simulink model "vexv5_Clawbot_Driver_Safety"  (R2019a)
settings: Solver=ode3  StartTime=0.0  StopTime=inf  RelTol=1e-3  EnableMultiTasking=on
libraries: vexv5lib x9, vexcommonlib x1
settings Model: ExtModeTrigDuration=5  Creator=The MathWorks, Inc.  LastModifiedBy=josea
settings DataIOCC: LimitDataPoints=on  SaveFormat=Array  ReturnWorkspaceOutputs=off
settings OptimizationCC: ExpressionDepthLimit=2147483647  LifeSpan=Inf  MaxStackSize=64
settings DebuggingCC: UnderspecifiedInitializationDetection=Classic  MergeDetectMultiDrivingBlocksExec=none  InheritedTsInSrcMsg=none  FcnCallInpInsideContextMsg=warning  UnconnectedInputMsg=none  UnconnectedOutputMsg=none  AllowSymbolicDim=off  StateNameClashWarn=warning  SFUnexpectedBacktrackingDiag=warning  SFNoUnconditionalDefaultTransitionDiag=warning  SFExecutionAtInitializationDiag=none  ArithmeticOperatorsInVariantConditions=warning
settings HardwareCC: ProdBitPerPointer=32  ProdBitPerSizeT=32  ProdBitPerPtrDiffT=32  ProdLargestAtomicInteger=Long  ProdLargestAtomicFloat=Double  ProdWordSize=32  ProdHWDeviceType=ARM Compatible->ARM Cortex
settings ModelReferenceCC: PropagateSignalLabelsOutOfModel=off
settings SFSimCC: SimUseLocalCustomCode=off
settings RTWCC: SystemTargetFile=ert.tlc  HardwareBoard=VEX V5 Robot Brain  TLCOptions=-aInlineSetEventsForThisBaseRateFcn=TLC_FALSE -aSuppressMultiTaskScheduler=TLC_FALSE -aRateBasedStepFcn=0  TemplateMakefile=ert_default_tmf  RTWUseLocalCustomCode=off  Toolchain=GNU Tools for ARM Embedded Processors
settings CodeAppCC: StateflowObjectComments=on
settings ERTTargetCC: CodeReplacementLibrary=GCC ARM Cortex-M3  MultiwordLength=2048  ERTCustomFileBanners=off  SupportContinuousTime=on  SupportNonInlinedSFcns=on  RemoveResetFunc=off  ModelStepFunctionPrototypeControlCompliant=off  ConvertIfToSwitch=off  SuppressUnreachableDefaultCases=off
settings ConfigComp: CovMetricSettings=dw  CovHtmlReporting=on  CovSaveCumulativeToWorkspaceVar=on  CovSaveSingleToWorkspaceVar=on  CovExternalEMLEnable=off  CovSFcnEnable=off

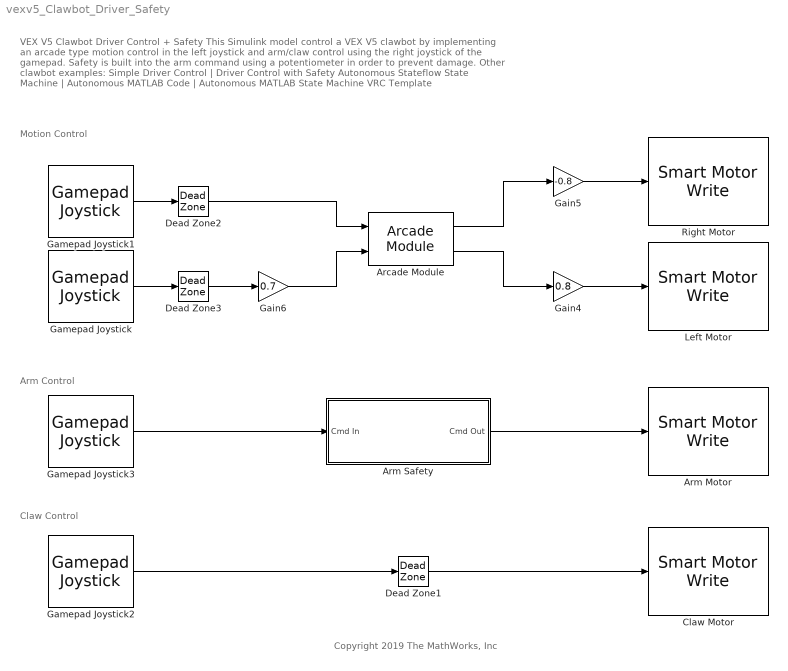
== system vexv5_Clawbot_Driver_Safety ==
  note: Claw Control
  note: Arm Control
  note: Motion Control
  note: Copyright 2019 The MathWorks, Inc
  note: VEX V5 Clawbot Driver Control + Safety
      | This Simulink model control a VEX V5 clawbot by implementing an arcade type motion control in the left joystick and arm/claw control using
      | the right joystick of the gamepad. Safety is built into the arm command using a potentiometer in order to prevent damage. Other clawbot examples:
      | Simple Driver Control | Driver Control with Safety
      | Autonomous Stateflow State Machine | Autonomous MATLAB Code | Autonomous MATLAB State Machine
      | VRC Template
  Arcade Module : vexcommonlib/Arcade Module  BlockPlatform=vexarmcortex
      settings: SourceProductName=Simulink Coder Support Package for ARM Cortex-based VEX Microcontroller  SourceProductBaseCode=EC_VEX_MICRO
  Arm Motor : vexv5lib/Actuators/Smart Motor Write  motorPort=8  scaleFactor=18:1  MotorBrakeMode=Hold  OperationMode=Velocity Control
      settings: SourceProductName=Simulink Coder Support Package for VEX EDR V5 Robot Brain
  Arm Safety : Subsystem
  Claw Motor : vexv5lib/Actuators/Smart Motor Write  motorPort=3  scaleFactor=18:1  MotorBrakeMode=Hold  OperationMode=Velocity Control
      settings: SourceProductName=Simulink Coder Support Package for VEX EDR V5 Robot Brain
  Dead Zone1 : DeadZone  LowerValue=-5  UpperValue=5  SaturateOnIntegerOverflow=on
  Dead Zone2 : DeadZone  LowerValue=-5  UpperValue=5  SaturateOnIntegerOverflow=on
  Dead Zone3 : DeadZone  LowerValue=-5  UpperValue=5  SaturateOnIntegerOverflow=on
  Gain4 : Gain  Gain=0.8
  Gain5 : Gain  Gain=-0.8
  Gain6 : Gain  Gain=0.7
  Gamepad Joystick : vexv5lib/Gamepad/Gamepad Joystick  joystickType=Master  chan=4  SampleTime=0.02
      settings: SourceProductName=Simulink Coder Support Package for VEX EDR V5 Robot Brain
  Gamepad Joystick1 : vexv5lib/Gamepad/Gamepad Joystick  joystickType=Master  chan=3  SampleTime=0.02
      settings: SourceProductName=Simulink Coder Support Package for VEX EDR V5 Robot Brain
  Gamepad Joystick2 : vexv5lib/Gamepad/Gamepad Joystick  joystickType=Master  chan=1  SampleTime=0.02
      settings: SourceProductName=Simulink Coder Support Package for VEX EDR V5 Robot Brain
  Gamepad Joystick3 : vexv5lib/Gamepad/Gamepad Joystick  joystickType=Master  chan=2  SampleTime=0.02
      settings: SourceProductName=Simulink Coder Support Package for VEX EDR V5 Robot Brain
  Left Motor : vexv5lib/Actuators/Smart Motor Write  motorPort=1  scaleFactor=18:1  MotorBrakeMode=Coast  OperationMode=Velocity Control
      settings: SourceProductName=Simulink Coder Support Package for VEX EDR V5 Robot Brain
  Right Motor : vexv5lib/Actuators/Smart Motor Write  motorPort=10  scaleFactor=18:1  MotorBrakeMode=Coast  OperationMode=Velocity Control
      settings: SourceProductName=Simulink Coder Support Package for VEX EDR V5 Robot Brain
  wires:
  Gamepad Joystick2/1 -> Dead Zone1/1
  Dead Zone3/1 -> Gain6/1
  Arcade Module/1 -> Gain5/1
  Arcade Module/2 -> Gain4/1
  Dead Zone2/1 -> Arcade Module/1
  Gain4/1 -> Left Motor/1
  Gamepad Joystick/1 -> Dead Zone3/1
  Gamepad Joystick1/1 -> Dead Zone2/1
  Gain5/1 -> Right Motor/1
  Gain6/1 -> Arcade Module/2
  Dead Zone1/1 -> Claw Motor/1
  Gamepad Joystick3/1 -> Arm Safety/1(Cmd In)
  Arm Safety/1(Cmd Out) -> Arm Motor/1

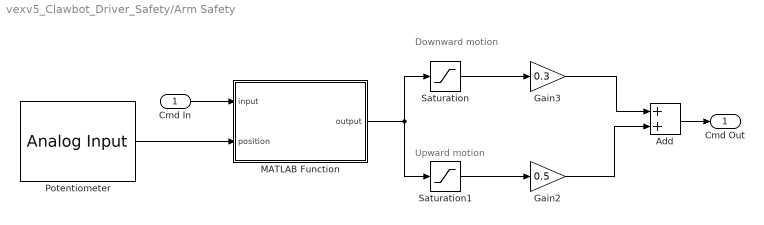
== system vexv5_Clawbot_Driver_Safety/Arm Safety ==
  note: Downward motion
  note: Upward motion
  Cmd In : Inport
  Add : Sum
  Gain2 : Gain  Gain=0.5
  Gain3 : Gain  Gain=0.3
  MATLAB Function : MATLAB Function  TreatAsAtomicUnit=on
  Potentiometer : vexv5lib/Sensors/Analog Input  port=A  SampleTime=0.02
      settings: SourceProductName=Simulink Coder Support Package for VEX EDR V5 Robot Brain
  Saturation : Saturate  UpperLimit=0  LowerLimit=-127
  Saturation1 : Saturate  UpperLimit=127  LowerLimit=0
  Cmd Out : Outport
  wires:
  Gain2/1 -> Add/2
  Add/1 -> Cmd Out/1
  Saturation/1 -> Gain3/1
  Saturation1/1 -> Gain2/1
  Gain3/1 -> Add/1
  MATLAB Function/1(output) -> Saturation/1, Saturation1/1
  Cmd In/1 -> MATLAB Function/1(input)
  Potentiometer/1 -> MATLAB Function/2(position)

== matlab function vexv5_Clawbot_Driver_Safety/Arm Safety/MATLAB Function ==
  data: input input; output output; position input
function output = armLimits(input, position)
% This MATLAB function limits the output sent to the clawbot arm motor
%  The output of this function is zero when the set maximum and minimum
%  potentiometer values are reached
if input >0 && position < 2650
    output=input;
elseif input <0 && position > 1400
    output=input;
else
    output=0;
end

end
